simulink model "MATLAB_TEST"  (R2019b)
(part 11 of 16)

  V_BCM_COM_DFCS_B_WOWs_Val_Acq/1 -> DTC16/1
  BCM_COM_PROC_P20/266 -> V_BCM_COM_A429_LMLG_Outboard_Tire_Press/1
  DTC90/1 -> BCM_COM_PROC_P20/90
  DTC15/1 -> BCM_COM_PROC_P20/15
  V_BCM_COM_DFCS_A_WOWs_Val_Acq/1 -> DTC15/1
  V_BCM_COM_DFCS_A_TLA_Above_Idle_Acq/1 -> DTC25/1
  V_BCM_COM_DFCS_B_NLG_WOWs_Acq/1 -> DTC14/1
  V_BCM_COM_Opt_Adhesion_In_Acq_W34/1 -> DTC75/1
  DTC14/1 -> BCM_COM_PROC_P20/14
  DTC13/1 -> BCM_COM_PROC_P20/13
  DTC73/1 -> BCM_COM_PROC_P20/73
  V_BCM_COM_DFCS_A_NLG_WOWs_Acq/1 -> DTC13/1
  BCM_COM_PROC_P20/133 -> V_BCM_COM_Whl_AS_Adp_Gain_W34/1
  DTC12/1 -> BCM_COM_PROC_P20/12
  BCM_COM_PROC_P20/161 -> V_BCM_COM_DFCS_B_Decel_Law_Inhib_Val/1
  DTC29/1 -> BCM_COM_PROC_P20/29
  BCM_COM_PROC_P20/663 -> Prb_FastStateCondition (2)/1  "Prb_FastStateCondition_2_BCMA"
  V_BCM_COM_LMLG_Downlock_Acq/1 -> DTC30/1
  DTC197/1 -> BCM_COM_PROC_P20/197
  DTC11/1 -> BCM_COM_PROC_P20/11
  BCM_COM_PROC_P20/439 -> Prb_RefSpeedLowLimit (2)/1  "Prb_RefSpeedLowLimit_7_BCMA"
  DTC10/1 -> BCM_COM_PROC_P20/10
  V_BCM_COM_DFCS_B_LMLG_WOWs_Acq/1 -> DTC10/1
  BCM_COM_PROC_P20/652 -> Prb_SoftSpeedResetOrder (2)/1  "Prb_SoftSpeedResetOrder_2_BCMA"
  DTC150/1 -> BCM_COM_PROC_P20/150
  DTC9/1 -> BCM_COM_PROC_P20/9
  DTC66/1 -> BCM_COM_PROC_P20/66
  BCM_COM_PROC_P20/154 -> V_BCM_COM_Hyd_B_Press_Conf_Flt/1
  DTC68/1 -> BCM_COM_PROC_P20/68
  DTC22/1 -> BCM_COM_PROC_P20/22
  DTC158/1 -> BCM_COM_PROC_P20/158
  BCM_COM_PROC_P20/855 -> v_BCM_COM_Regular_Brkg_Press_Cmd/1  "v_BCM_COM_Regular_Brkg_Press_Cmd_1_BCMA"
  DTC26/1 -> BCM_COM_PROC_P20/26
  DTC27/1 -> BCM_COM_PROC_P20/27
  V_BCM_COM_DFCS_A_LMLG_WOWs_Acq/1 -> DTC9/1
  V_BCM_COM_PBSELV_ON_POS_Unconf_Flt/1 -> DTC54/1
  BCM_COM_PROC_P20/541 -> Prb_SoftSpeedCountOrder/1  "Prb_SoftSpeedCountOrder_4_BCMA"
  V_BCM_COM_DFCS_B_Pitch_Ang_Acq/1 -> DTC8/1
  DTC220/1 -> BCM_COM_PROC_P20/220
  V_BCM_COM_DFCS_A_Pitch_Ang_Acq/1 -> DTC7/1
  V_BCM_COM_LMLG_Dnlk_Unconf_Flt/1 -> DTC32/1
  DTC32/1 -> BCM_COM_PROC_P20/32
  V_BCM_COM_DFCS_B_Long_Accel_Acq/1 -> DTC6/1
  BCM_COM_PROC_P20/9 -> V_BCM_COM_DFCS_A_Long_Accel_Conv/1
  DTC208/1 -> BCM_COM_PROC_P20/208
  V_BCM_COM_PBSELV_ON_POS_Conf_Flt/1 -> DTC55/1
  BCM_COM_PROC_P20/857 -> PRB_RateLimitation/1  "PRB_RateLimitation_2_BCMA"
  DTC6/1 -> BCM_COM_PROC_P20/6
  DTC155/1 -> BCM_COM_PROC_P20/155
  DTC19/1 -> BCM_COM_PROC_P20/19
  DTC5/1 -> BCM_COM_PROC_P20/5
  V_BCM_COM_Norm_Brkg_Off_Sanc/1 -> DTC48/1
  V_BCM_COM_DFCS_B_RMLG_WOWs_Acq/1 -> DTC12/1
  V_BCM_COM_CF_DBCU_FAILED/1 -> DTC50/1
  BCM_COM_PROC_P20/84 -> V_BCM_COM_RH_Eng_Run_Press_Cmd/1
  V_BCM_COM_DFCS_A_Long_Accel_Acq/1 -> DTC5/1
  BCM_COM_PROC_P20/396 -> V_BCM_COM_ETH_FB_LMLG_DWNLOCK_FAIL/1
  V_BCM_COM_Whl_LP_AS_Curr_Order_W12/1 -> DTC66/1
  DTC4/1 -> BCM_COM_PROC_P20/4
  BCM_COM_PROC_P20/181 -> V_BCM_COM_DFCS_A_TLA_Above_Idle_Val/1
  V_BCM_COM_DFCS_B_Gnd_Spd_Acq/1 -> DTC4/1
  V_BCM_COM_DFCS_A_RMLG_WOWs_Acq/1 -> DTC11/1
  DTC3/1 -> BCM_COM_PROC_P20/3
  DTC2/1 -> BCM_COM_PROC_P20/2
  DTC7/1 -> BCM_COM_PROC_P20/7
  BCM_COM_PROC_P20/1 -> V_BCM_COM_Whl_Spun_Up_State_W12/1
  BCM_COM_PROC_P20/824 -> v_BCM_COM_UF_DFCS_B_RMLGWOW_1_RX/1  "v_BCM_COM_UF_DFCS_B_RMLGWOW_1_RX_1_BCMA"
  DTC1/1 -> BCM_COM_PROC_P20/1
  DTC216/1 -> BCM_COM_PROC_P20/216
  V_BCM_COM_Tacho_Conf_Flt_W34/1 -> DTC2/1
  DTC215/1 -> BCM_COM_PROC_P20/215
  DTC8/1 -> BCM_COM_PROC_P20/8
  V_BCM_COM_DFCS_A_Gnd_Spd_Acq/1 -> DTC3/1
  BCM_COM_PROC_P20/467 -> Prb_OnGroundAfterHydroTransition (3)/1  "Prb_OnGroundAfterHydroTransition_1_BCMA"
  V_BCM_COM_Tacho_Conf_Flt_W12/1 -> DTC1/1
  V_BCM_COM_LG_Lever_Up_Conf_Flt/1 -> DTC29/1
  BCM_Tuning/1 -> Subsystem/1(In1)
  Subsystem/1(Out1) -> BCM_COM_PROC_P20/230
  Subsystem/2(Out2) -> BCM_COM_PROC_P20/231
  Subsystem/3(Out3) -> BCM_COM_PROC_P20/232
  Subsystem/4(Out4) -> BCM_COM_PROC_P20/233
  Subsystem/5(Out5) -> BCM_COM_PROC_P20/234
  Subsystem/6(Out6) -> BCM_COM_PROC_P20/235
  Subsystem/7(Out7) -> BCM_COM_PROC_P20/236
  Subsystem/8(Out8) -> BCM_COM_PROC_P20/237
  Subsystem/9(Out9) -> BCM_COM_PROC_P20/238
  Subsystem/10(Out10) -> BCM_COM_PROC_P20/239
  Subsystem/11(Out11) -> BCM_COM_PROC_P20/240
  Subsystem/12(Out12) -> BCM_COM_PROC_P20/241
  Subsystem/13(Out13) -> BCM_COM_PROC_P20/242
  Subsystem/14(Out14) -> BCM_COM_PROC_P20/243
  Subsystem/15(Out15) -> BCM_COM_PROC_P20/244
  Subsystem/16(Out16) -> BCM_COM_PROC_P20/245
  Subsystem/17(Out17) -> BCM_COM_PROC_P20/246
  Subsystem/18(Out18) -> BCM_COM_PROC_P20/247
  Subsystem/19(Out19) -> BCM_COM_PROC_P20/248
  Subsystem/20(Out20) -> BCM_COM_PROC_P20/249
  Subsystem/21(Out21) -> BCM_COM_PROC_P20/250
  Subsystem/22(Out22) -> BCM_COM_PROC_P20/251
  Subsystem/23(Out23) -> BCM_COM_PROC_P20/252
  Subsystem/24(Out24) -> BCM_COM_PROC_P20/253
  Subsystem/25(Out25) -> BCM_COM_PROC_P20/254
  Subsystem/26(Out26) -> BCM_COM_PROC_P20/255
  Subsystem/27(Out27) -> BCM_COM_PROC_P20/256
  Subsystem/28(Out28) -> BCM_COM_PROC_P20/257
  Subsystem/29(Out29) -> BCM_COM_PROC_P20/258
  Subsystem/30(Out30) -> BCM_COM_PROC_P20/259
  Subsystem/31(Out31) -> BCM_COM_PROC_P20/260
  Subsystem/32(Out32) -> BCM_COM_PROC_P20/261
  Subsystem/33(Out33) -> BCM_COM_PROC_P20/262
  Subsystem/34(Out34) -> BCM_COM_PROC_P20/263
  Subsystem/35(Out35) -> BCM_COM_PROC_P20/264
  Subsystem/36(Out36) -> BCM_COM_PROC_P20/265
  Subsystem/37(Out37) -> BCM_COM_PROC_P20/266
  Subsystem/38(Out38) -> BCM_COM_PROC_P20/267
  Subsystem/39(Out39) -> BCM_COM_PROC_P20/268
  Subsystem/40(Out40) -> BCM_COM_PROC_P20/269
  Subsystem/41(Out41) -> BCM_COM_PROC_P20/270
  Subsystem/42(Out42) -> BCM_COM_PROC_P20/271
  Subsystem/43(Out43) -> BCM_COM_PROC_P20/272
  Subsystem/44(Out44) -> BCM_COM_PROC_P20/273
  Subsystem/45(Out45) -> BCM_COM_PROC_P20/274
  Subsystem/46(Out46) -> BCM_COM_PROC_P20/275
  Subsystem/47(Out47) -> BCM_COM_PROC_P20/276
  Subsystem/48(Out48) -> BCM_COM_PROC_P20/277
  Subsystem/49(Out49) -> BCM_COM_PROC_P20/278
  Subsystem/50(Out50) -> BCM_COM_PROC_P20/279
  Subsystem/51(Out51) -> BCM_COM_PROC_P20/280
  Subsystem/52(Out52) -> BCM_COM_PROC_P20/281
  Subsystem/53(Out53) -> BCM_COM_PROC_P20/282
  Subsystem/54(Out54) -> BCM_COM_PROC_P20/283
  Subsystem/55(Out55) -> BCM_COM_PROC_P20/284
  Subsystem/56(Out56) -> BCM_COM_PROC_P20/285
  Subsystem/57(Out57) -> BCM_COM_PROC_P20/286
  Subsystem/58(Out58) -> BCM_COM_PROC_P20/287
  Subsystem/59(Out59) -> BCM_COM_PROC_P20/288
  Subsystem/60(Out60) -> BCM_COM_PROC_P20/289
  Subsystem/61(Out61) -> BCM_COM_PROC_P20/290
  Subsystem/62(Out62) -> BCM_COM_PROC_P20/291
  Subsystem/63(Out63) -> BCM_COM_PROC_P20/292
  Subsystem/64(Out64) -> BCM_COM_PROC_P20/293
  Subsystem/65(Out65) -> BCM_COM_PROC_P20/294
  Subsystem/66(Out66) -> BCM_COM_PROC_P20/295
  Subsystem/67(Out67) -> BCM_COM_PROC_P20/296
  Subsystem/68(Out68) -> BCM_COM_PROC_P20/297
  Subsystem/69(Out69) -> BCM_COM_PROC_P20/298
  Subsystem/70(Out70) -> BCM_COM_PROC_P20/299
  Subsystem/71(Out71) -> BCM_COM_PROC_P20/300
  Subsystem/72(Out72) -> BCM_COM_PROC_P20/301
  Subsystem/73(Out73) -> BCM_COM_PROC_P20/302
  Subsystem/74(Out74) -> BCM_COM_PROC_P20/303
  Subsystem/75(Out75) -> BCM_COM_PROC_P20/304
  Subsystem/76(Out76) -> BCM_COM_PROC_P20/305
  Subsystem/77(Out77) -> BCM_COM_PROC_P20/306
  Subsystem/78(Out78) -> BCM_COM_PROC_P20/307
  Subsystem/79(Out79) -> BCM_COM_PROC_P20/308
  Subsystem/80(Out80) -> BCM_COM_PROC_P20/309
  Subsystem/81(Out81) -> BCM_COM_PROC_P20/310
  Subsystem/82(Out82) -> BCM_COM_PROC_P20/311
  Subsystem/83(Out83) -> BCM_COM_PROC_P20/312
  Subsystem/84(Out84) -> BCM_COM_PROC_P20/313
  Subsystem/85(Out85) -> BCM_COM_PROC_P20/314
  Subsystem/86(Out86) -> BCM_COM_PROC_P20/315
  Subsystem/87(Out87) -> BCM_COM_PROC_P20/316
  Subsystem/88(Out88) -> BCM_COM_PROC_P20/317
  Subsystem/89(Out89) -> BCM_COM_PROC_P20/318
  Subsystem/90(Out90) -> BCM_COM_PROC_P20/319
  Subsystem/91(Out91) -> BCM_COM_PROC_P20/320
  Subsystem/92(Out92) -> BCM_COM_PROC_P20/321
  Subsystem/93(Out93) -> BCM_COM_PROC_P20/322
  Subsystem/94(Out94) -> BCM_COM_PROC_P20/323
  Subsystem/95(Out95) -> BCM_COM_PROC_P20/324
  Subsystem/96(Out96) -> BCM_COM_PROC_P20/325
  Subsystem/97(Out97) -> BCM_COM_PROC_P20/326
  Subsystem/98(Out98) -> BCM_COM_PROC_P20/327
  Subsystem/99(Out99) -> BCM_COM_PROC_P20/328
  Subsystem/100(Out100) -> BCM_COM_PROC_P20/329
  Subsystem/101(Out101) -> BCM_COM_PROC_P20/330
  Subsystem/102(Out102) -> BCM_COM_PROC_P20/331
  Subsystem/103(Out103) -> BCM_COM_PROC_P20/332
  Subsystem/104(Out104) -> BCM_COM_PROC_P20/333
  Subsystem/105(Out105) -> BCM_COM_PROC_P20/334
  Subsystem/106(Out106) -> BCM_COM_PROC_P20/335
  Subsystem/107(Out107) -> BCM_COM_PROC_P20/336
  Subsystem/108(Out108) -> BCM_COM_PROC_P20/337
  Subsystem/109(Out109) -> BCM_COM_PROC_P20/338
  Subsystem/110(Out110) -> BCM_COM_PROC_P20/339
  Subsystem/111(Out111) -> BCM_COM_PROC_P20/340
  Subsystem/112(Out112) -> BCM_COM_PROC_P20/341
  Subsystem/113(Out113) -> BCM_COM_PROC_P20/342
  Subsystem/114(Out114) -> BCM_COM_PROC_P20/343
  Subsystem/115(Out115) -> BCM_COM_PROC_P20/344
  Subsystem/116(Out116) -> BCM_COM_PROC_P20/345
  Subsystem/117(Out117) -> BCM_COM_PROC_P20/346
  Subsystem/118(Out118) -> BCM_COM_PROC_P20/347
  Subsystem/119(Out119) -> BCM_COM_PROC_P20/348
  Subsystem/120(Out120) -> BCM_COM_PROC_P20/349
  Subsystem/121(Out121) -> BCM_COM_PROC_P20/350
  Subsystem/122(Out122) -> BCM_COM_PROC_P20/351
  Subsystem/123(Out123) -> BCM_COM_PROC_P20/352
  Subsystem/124(Out124) -> BCM_COM_PROC_P20/353
  Subsystem/125(Out125) -> BCM_COM_PROC_P20/354
  Subsystem/126(Out126) -> BCM_COM_PROC_P20/355
  Subsystem/127(Out127) -> BCM_COM_PROC_P20/356
  Subsystem/128(Out128) -> BCM_COM_PROC_P20/357
  Subsystem/129(Out129) -> BCM_COM_PROC_P20/358
  Subsystem/130(Out130) -> BCM_COM_PROC_P20/359
  Subsystem/131(Out131) -> BCM_COM_PROC_P20/360
  Subsystem/132(Out132) -> BCM_COM_PROC_P20/361
  Subsystem/133(Out133) -> BCM_COM_PROC_P20/362
  Subsystem/134(Out134) -> BCM_COM_PROC_P20/363
  Subsystem/135(Out135) -> BCM_COM_PROC_P20/364
  Subsystem/136(Out136) -> BCM_COM_PROC_P20/365
  Subsystem/137(Out137) -> BCM_COM_PROC_P20/366
  Subsystem/138(Out138) -> BCM_COM_PROC_P20/367
  Subsystem/139(Out139) -> BCM_COM_PROC_P20/368
  Subsystem/140(Out140) -> BCM_COM_PROC_P20/369
  Subsystem/141(Out141) -> BCM_COM_PROC_P20/370
  Subsystem/142(Out142) -> BCM_COM_PROC_P20/371
  Subsystem/143(Out143) -> BCM_COM_PROC_P20/372
  Subsystem/144(Out144) -> BCM_COM_PROC_P20/373
